simulink subsystem "WinchController"  (R2021a)
settings: Solver=VariableStepAuto  StartTime=0.0  StopTime=10.0  RelTol=1e-3
settings Model: Creator=ufechner  LastModifiedBy=ufechner

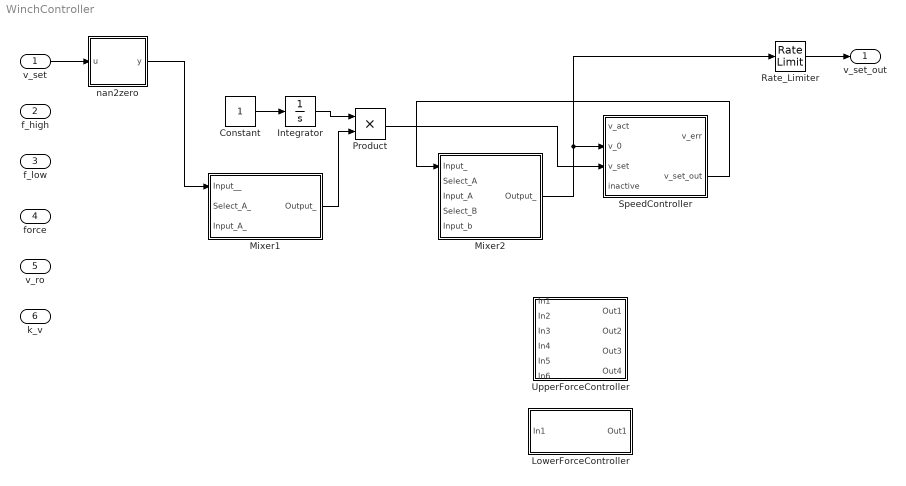
== system WinchController ==
  v_set : Inport
  f_high : Inport  Port=2
  f_low : Inport  Port=3
  force : Inport  Port=4
  v_ro : Inport  Port=5
  k_v : Inport  Port=6
  Constant : Constant
  Integrator : Integrator  LimitOutput=on  UpperSaturationLimit=1  LowerSaturationLimit=0
  LowerForceController : Subsystem
  Mixer1 : Subsystem
  Mixer2 : Subsystem
  Product : Product
  Rate_Limiter : RateLimiter  SampleTimeMode=inherited
  SpeedController : Subsystem
  UpperForceController : Subsystem
  nan2zero : MATLAB Function  TreatAsAtomicUnit=on
  v_set_out : Outport
  wires:
  Rate_Limiter/1 -> v_set_out/1
  SpeedController/2(v_set_out) -> Mixer2/1(Input_)
  Mixer2/1(Output_) -> SpeedController/2(v_0), Rate_Limiter/1
  v_set/1 -> nan2zero/1(u)
  nan2zero/1(y) -> Mixer1/1(Input__)
  Constant/1 -> Integrator/1
  Integrator/1 -> Product/1
  Mixer1/1(Output_) -> Product/2
  Product/1 -> SpeedController/3(v_set)

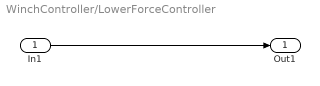
== system WinchController/LowerForceController ==
  In1 : Inport
  Out1 : Outport
  wires:
  In1/1 -> Out1/1

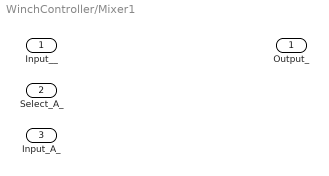
== system WinchController/Mixer1 ==
  Input__ : Inport
  Select_A_ : Inport  Port=2
  Input_A_ : Inport  Port=3
  Output_ : Outport

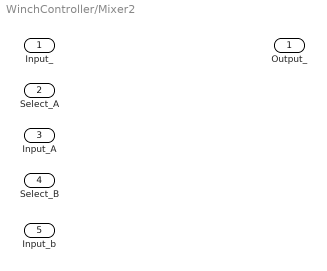
== system WinchController/Mixer2 ==
  Input_ : Inport
  Select_A : Inport  Port=2
  Input_A : Inport  Port=3
  Select_B : Inport  Port=4
  Input_b : Inport  Port=5
  Output_ : Outport

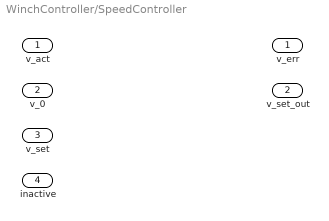
== system WinchController/SpeedController ==
  v_act : Inport
  v_0 : Inport  Port=2
  v_set : Inport  Port=3
  inactive : Inport  Port=4
  v_err : Outport
  v_set_out : Outport  Port=2

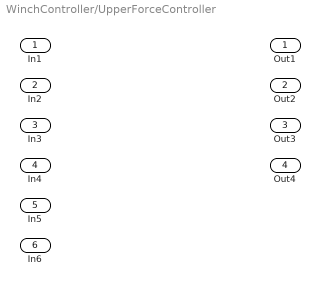
== system WinchController/UpperForceController ==
  In1 : Inport
  In2 : Inport  Port=2
  In3 : Inport  Port=3
  In4 : Inport  Port=4
  In5 : Inport  Port=5
  In6 : Inport  Port=6
  Out1 : Outport
  Out2 : Outport  Port=2
  Out3 : Outport  Port=3
  Out4 : Outport  Port=4

== matlab function WinchController/nan2zero ==
  data: u input; y output
function y = fcn(u)
%#codegen

y = u;
